simulink model "my"  (R2021a)
settings: Solver=VariableStepAuto  StartTime=0.0  StopTime=20  RelTol=1e-3
model workspace (MAT data in the model file):
  tc = 0.01
values from neighbouring files (symbols this model uses):
  cf = -155016    [emplanner_init.m]
  cr = -92204    [emplanner_init.m]
  la = 1.225    [emplanner_init.m]
  lb = 2.68-1.225    (= 1.455)    [emplanner_init.m]    (also in la3.m = -0.6; mpc_speed_control.m = kron(ones(Nc,1),-dumax))
  LQR_K1 = k(:,1)'    [emplanner_init.m]
  LQR_K2 = k(:,2)'    [emplanner_init.m]
  LQR_K3 = k(:,3)'    [emplanner_init.m]
  LQR_K4 = k(:,4)'    [emplanner_init.m]
  m = VehConf.m    [GetMPCControlMatrix.m]    (also in emplanner_init.m = 1422; getcontrol.m)
  vx_break_point = zeros(1,5000)    [emplanner_init.m]
libraries: simulink x3, pid_lib x2, Solver_SF x1
settings Model: Creator=t  LastModifiedBy=t

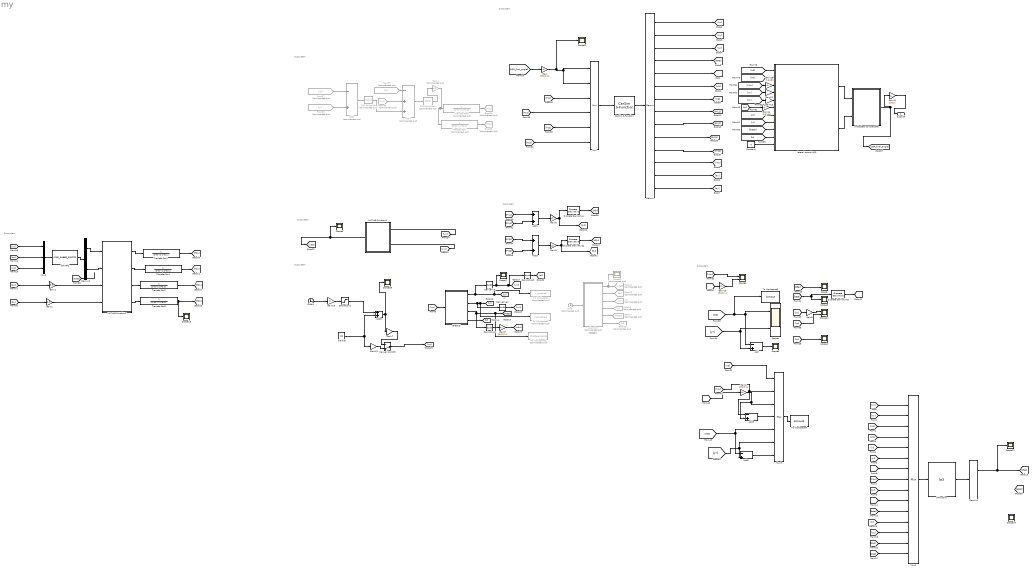
== system my ==
  note: Subsystem
  note: Subsystem
  note: Subsystem
  note: Subsystem
  note: Subsystem
  note: Subsystem
  note: 规划接口
  note: Subsystem
  Add : Sum  Inputs=-+
  Add1 : Sum
  Add2 : Sum  Commented=on  Inputs=-+
  Add3 : Sum
  Add4 : Sum  Commented=on  Inputs=-++
  Add5 : Sum  Inputs=-+
  Add6 : Sum  Inputs=-+
  Add8 : Sum
  CarSim S-Function : Solver_SF/CarSim S-Function  Priority=1  SIMFILE=simfile.sim  Run_RTs=off  vs_state_ind=Run  StopMode_ind=Vehicle Model
  Clock : Clock  Commented=on
  Clock1 : Clock
  Constant : Constant  Value=0
  Demux : Demux  Outputs=14
  Demux1 : Demux  Outputs=2
  Demux2 : Demux  Outputs=2
  Derivative{,1..3} (4 alike) : Derivative
  Discrete Derivative : simulink/Discrete/Discrete Derivative  gainval=1.0  ICPrevScaledInput=0.0  OutMin=[]  OutMax=[]  OutDataType=fixdt(1, 16)  OutScaling=2^-10  DoSatur=off
  Discrete Derivative1 : simulink/Discrete/Discrete Derivative  gainval=1.0  ICPrevScaledInput=0.0  OutMin=[]  OutMax=[]  OutDataType=fixdt(1, 16)  OutScaling=2^-10  DoSatur=off
  Discrete Derivative2 : simulink/Discrete/Discrete Derivative  gainval=1.0  ICPrevScaledInput=0.0  OutMin=[]  OutMax=[]  OutDataType=fixdt(1, 16)  OutScaling=2^-10  DoSatur=off
  From37 : From  Commented=on  GotoTag=xO
  From38 : From  Commented=on  GotoTag=xr
  From39 : From  Commented=on  GotoTag=Vx
  From46 : From  Commented=on  GotoTag=vp
  Gain{,3,6,10} (4 alike) : Gain  Gain=180/3.14
  Gain1 : Gain  Gain=9.8
  Gain11 : Gain  Gain=180/pi
  Gain{5,7,12..13,20} (5 alike) : Gain  Gain=1/3.6
  Gain14 : Gain  Gain=3.6/180
  Gain15 : Gain  Gain=3.6/180
  Gain19 : Gain  Gain=2
  Gain2 : Gain  Gain=9.8
  Gain4 : Gain  Commented=on  Gain=1/2
  Gain8 : Gain  Gain=1/2
  Gain9 : Gain  Gain=1/2
  Goto16 : Goto  Commented=on  GotoTag=yr
  Goto17 : Goto  Commented=on  GotoTag=thetar
  Goto18 : Goto  Commented=on  GotoTag=kr
  Goto24 : Goto  Commented=on  GotoTag=vdes
  Goto25 : Goto  Commented=on  GotoTag=ar
  Goto34 : Goto  Commented=on  GotoTag=T21
  Goto35 : Goto  Commented=on  GotoTag=T22
  MATLAB Function1 : MATLAB Function  TreatAsAtomicUnit=on
  MATLAB Function2 : MATLAB Function  TreatAsAtomicUnit=on
  Manual Switch5 : ManualSwitch  CurrentSetting=0
  Mux : Mux  Inputs=6
  Mux1 : Mux  Inputs=15
  Mux2 : Mux  Inputs=3
  Mux3 : Mux  Inputs=7
  PID Controller : pid_lib/PID Controller  Commented=on  Controller=PID  Form=Parallel  TimeDomain=Continuous-time  UseExternalTs=off  SampleTime=-1  IntegratorMethod=Forward Euler  FilterMethod=Forward Euler  ControllerParametersSource=internal  P=1  I=0.01  D=0  UseFilter=on  N=100  TunerSelectOption=Transfer Function Based (PID Tuner App)  InitialConditionSource=internal  InitialConditionForIntegrator=0  InitialConditionForFilter=0  DifferentiatorICPrevScaledInput=0  ExternalReset=none  TrackingMode=off  Kt=1  LimitOutput=off  SatLimitsSource=internal  UpperSaturationLimit=inf  LowerSaturationLimit=-inf  LinearizeAsGain=on  AntiWindupMode=none  Kb=1  POutMin=[]  POutMax=[]  IOutMin=[]  IOutMax=[]  DOutMin=[]  DOutMax=[]  NOutMin=[]  NOutMax=[]  SumOutMin=[]  SumOutMax=[]  SaturationOutMin=[]  SaturationOutMax=[]  PParamMin=[]  PParamMax=[]  IParamMin=[]  IParamMax=[]  DParamMin=[]  DParamMax=[]  NParamMin=[]  NParamMax=[]  KbParamMin=[]  KbParamMax=[]  KtParamMin=[]  KtParamMax=[]  KbOutMin=[]  KbOutMax=[]  KtOutMin=[]  KtOutMax=[]  IntegratorOutMin=[]  IntegratorOutMax=[]  FilterOutMin=[]  FilterOutMax=[]  SumI1OutMin=[]  SumI1OutMax=[]  SumI2OutMin=[]  SumI2OutMax=[]  SumI3OutMin=[]  SumI3OutMax=[]  SumI4OutMin=[]  SumI4OutMax=[]  SumDOutMin=[]  SumDOutMax=[]  DifferentiatorOutMin=[]  DifferentiatorOutMax=[]  FilterDiffOutCoefMin=[]  FilterDiffOutCoefMax=[]  ReciprocalOutMin=[]  ReciprocalOutMax=[]  SumDenOutMin=[]  SumDenOutMax=[]  SumNumOutMin=[]  SumNumOutMax=[]  DivideOutMin=[]  DivideOutMax=[]  UdiffTsProdOutMin=[]  UdiffTsProdOutMax=[]  NTsProdOutMin=[]  NTsProdOutMax=[]  UintegralTsProdOutMin=[]  UintegralTsProdOutMax=[]  UngainTsProdOutMin=[]  UngainTsProdOutMax=[]  IntegratorContinuousStateAttributes=''  IntegratorStateMustResolveToSignalObject=off  IntegratorRTWStateStorageClass=Auto  FilterContinuousStateAttributes=''  FilterStateMustResolveToSignalObject=off  FilterRTWStateStorageClass=Auto  ParallelPVariant=InternalParameters  IdealPVariant=Disabled  IVariant=InternalParameters  DVariant=InternalParameters  IntegratorVariant=Continuous  SatVariant=Disabled  AWVariant=Passthrough  PCopyVariant=Disabled  TRVariant=Disabled  FdbkBlocksVariant=Forward  IdealPFdbkVariant=Disabled  SatFdbkVariant=Disabled  DerivativeFilterVariant=ContFilter  NVariant=InternalParameters  NCopyVariant=Disabled  FilterICVariant=InternalICsFilter  IntegratorICVariant=InternalICs  ExternalResetVariant=Disabled  TRSumVariant=Passthrough  SumFdbkVariant=Disabled  SumVariant=Sum_PID  TsampFilterVariant=InternalTs  TsampNgainVariant=Passthrough  TsampIntegralVariant=Passthrough  ExternalSaturationOutDataTypeStr=Inherit: Same as second input
  PID Controller1 : pid_lib/PID Controller  Commented=on  Controller=PID  Form=Parallel  TimeDomain=Continuous-time  UseExternalTs=off  SampleTime=-1  IntegratorMethod=Forward Euler  FilterMethod=Forward Euler  ControllerParametersSource=internal  P=0.03  I=0.2  D=0  UseFilter=on  N=100  TunerSelectOption=Transfer Function Based (PID Tuner App)  InitialConditionSource=internal  InitialConditionForIntegrator=0  InitialConditionForFilter=0  DifferentiatorICPrevScaledInput=0  ExternalReset=none  TrackingMode=off  Kt=1  LimitOutput=off  SatLimitsSource=internal  UpperSaturationLimit=inf  LowerSaturationLimit=-inf  LinearizeAsGain=on  AntiWindupMode=none  Kb=1  POutMin=[]  POutMax=[]  IOutMin=[]  IOutMax=[]  DOutMin=[]  DOutMax=[]  NOutMin=[]  NOutMax=[]  SumOutMin=[]  SumOutMax=[]  SaturationOutMin=[]  SaturationOutMax=[]  PParamMin=[]  PParamMax=[]  IParamMin=[]  IParamMax=[]  DParamMin=[]  DParamMax=[]  NParamMin=[]  NParamMax=[]  KbParamMin=[]  KbParamMax=[]  KtParamMin=[]  KtParamMax=[]  KbOutMin=[]  KbOutMax=[]  KtOutMin=[]  KtOutMax=[]  IntegratorOutMin=[]  IntegratorOutMax=[]  FilterOutMin=[]  FilterOutMax=[]  SumI1OutMin=[]  SumI1OutMax=[]  SumI2OutMin=[]  SumI2OutMax=[]  SumI3OutMin=[]  SumI3OutMax=[]  SumI4OutMin=[]  SumI4OutMax=[]  SumDOutMin=[]  SumDOutMax=[]  DifferentiatorOutMin=[]  DifferentiatorOutMax=[]  FilterDiffOutCoefMin=[]  FilterDiffOutCoefMax=[]  ReciprocalOutMin=[]  ReciprocalOutMax=[]  SumDenOutMin=[]  SumDenOutMax=[]  SumNumOutMin=[]  SumNumOutMax=[]  DivideOutMin=[]  DivideOutMax=[]  UdiffTsProdOutMin=[]  UdiffTsProdOutMax=[]  NTsProdOutMin=[]  NTsProdOutMax=[]  UintegralTsProdOutMin=[]  UintegralTsProdOutMax=[]  UngainTsProdOutMin=[]  UngainTsProdOutMax=[]  IntegratorContinuousStateAttributes=''  IntegratorStateMustResolveToSignalObject=off  IntegratorRTWStateStorageClass=Auto  FilterContinuousStateAttributes=''  FilterStateMustResolveToSignalObject=off  FilterRTWStateStorageClass=Auto  ParallelPVariant=InternalParameters  IdealPVariant=Disabled  IVariant=InternalParameters  DVariant=InternalParameters  IntegratorVariant=Continuous  SatVariant=Disabled  AWVariant=Passthrough  PCopyVariant=Disabled  TRVariant=Disabled  FdbkBlocksVariant=Forward  IdealPFdbkVariant=Disabled  SatFdbkVariant=Disabled  DerivativeFilterVariant=ContFilter  NVariant=InternalParameters  NCopyVariant=Disabled  FilterICVariant=InternalICsFilter  IntegratorICVariant=InternalICs  ExternalResetVariant=Disabled  TRSumVariant=Passthrough  SumFdbkVariant=Disabled  SumVariant=Sum_PID  TsampFilterVariant=InternalTs  TsampNgainVariant=Passthrough  TsampIntegralVariant=Passthrough  ExternalSaturationOutDataTypeStr=Inherit: Same as second input
  S-Function : S-Function  FunctionName=la3  SFunctionDeploymentMode=off  EnableBusSupport=off
  Saturation1 : Saturate  UpperLimit=18  LowerLimit=-18
  Scope{,1,3,5..8,10,12..13,28} (11 alike) : Scope
  Scope11 : Scope  NumInputPorts=2
  Scope2 : Scope  NumInputPorts=2
  Scope4 : Scope  NumInputPorts=2
  Scope9 : Scope  Commented=on
  To Workspace : ToWorkspace  Commented=on  VariableName=x_experice  SaveFormat=Timeseries  SampleTime=-1
  To Workspace1 : ToWorkspace  Commented=on  VariableName=y_experice1  SaveFormat=Timeseries  SampleTime=-1
  To Workspace2 : ToWorkspace  Commented=on  VariableName=theate_experice  SaveFormat=Timeseries  SampleTime=-1
  To Workspace3 : ToWorkspace  VariableName=simout  SaveFormat=Timeseries  SampleTime=-1
  To Workspace4 : ToWorkspace  VariableName=simout1  SaveFormat=Timeseries  SampleTime=-1
  Transfer Fcn{1..4} (4 alike) : TransferFcn  Denominator=[2*tc^2 2*tc 1]
  Transfer Fcn6 : TransferFcn  Commented=on  Denominator=[2*tc^2 2*tc 1]
  Transfer Fcn7 : TransferFcn  Commented=on  Denominator=[2*tc^2 2*tc 1]
  lateral control LQR : Subsystem
  planning : MATLAB Function  Commented=on  TreatAsAtomicUnit=on
  understeer compensate : Subsystem
  xr1 : Goto  Commented=on  GotoTag=xr
  参考轨迹 : Subsystem
  目标车速 : Constant  Value=60
  纵向MPC : S-Function  FunctionName=mpc_speed_control  SFunctionDeploymentMode=off  EnableBusSupport=off
  Output3 : Outport
  wires:
  ? -> [ades], Scope10/1
  planning/6(kr) -> Goto18/1  "曲率"
  [xO] -> lateral control LQR/1(host_x[m])
  Demux/7 -> [YO]
  [yr] -> lateral control LQR/8(yr)
  [ax] -> Gain1/1
  Gain14/1 -> lateral control LQR/6(host_yaw_dot[rad/s])
  lateral control LQR/1(Output) -> understeer compensate/1(LQR_angle)
  Transfer Fcn4/1 -> [T11]
  Add4/1 -> PID Controller1/1
  Gain12/1 -> lateral control LQR/4(host_vx[m/s])
  Discrete Derivative1/1 -> [dfyr]
  [Vx] -> Gain12/1
  [vp] -> Scope11/2
  [bata] -> Mux1/11
  Gain10/1 -> Scope2/2
  PID Controller1/1 -> Gain4/1
  PID Controller/1 -> Add4/3
  [CAF] -> Mux1/14
  [FYL1] -> Add1/1
  [kr] -> lateral control LQR/10(kappar)
  Demux/8 -> [FYL1]  "FYL1"
  Add2/1 -> PID Controller/1
  From39/1 -> Add4/1
  MATLAB Function2/4(T22) -> Transfer Fcn3/1
  From38/1 -> Add2/2
  Derivative3/1 -> [ar]
  From46/1 -> Add4/2
  From37/1 -> Add2/1
  Gain1/1 -> MATLAB Function2/3(ax)
  Demux/14 -> [ay]  "横向加速度"
  [LQR_final_angle] -> Gain/1  "转角"
  Demux/3 -> [wr]  "横摆角速度deg/s"
  [wr] -> Mux1/9
  [yr] -> Add/2, Scope4/2
  [xr] -> Mux1/5
  lateral control LQR/2(Output1) -> understeer compensate/2(lateral err)
  [T11] -> Mux/3
  [YO] -> To Workspace3/1, Scope4/1, Add/1
  Demux/12 -> [YAw]  "ya(deg)"
  [T22] -> Mux/6
  [dbate] -> Mux1/10
  [YAw] -> Mux1/8
  Demux/1 -> [Vx]  "vx(km/h)"
  [T12] -> Mux/4
  [vp] -> Mux2/3
  [Vx] -> Gain5/1
  Gain3/1 -> [wthr]
  [stter] -> Scope/1
  [wr] -> Scope1/1
  Transfer Fcn2/1 -> [T21]
  Mux2/1 -> 纵向MPC/1
  MATLAB Function2/1(T11) -> Transfer Fcn4/1
  目标车速/1 -> Gain20/1, Add8/2
  Gain20/1 -> Manual Switch5/2
  Clock1/1 -> Gain19/1
  参考轨迹/3(yawr) -> Derivative2/1, To Workspace2/1, [thetar]  "yawa"
  planning/4(yr) -> Goto16/1
  Gain19/1 -> Saturation1/1
  Saturation1/1 -> Add8/1
  Manual Switch5/1 -> [vp]
  Gain7/1 -> Manual Switch5/1
  Add8/1 -> Gain7/1, Scope28/1
  planning/2(ap) -> Goto25/1  "ap"
  [ades] -> ?
  参考轨迹/2(yr) -> Derivative1/1, To Workspace1/1, [yr]
  MATLAB Function2/3(T21) -> Transfer Fcn2/1
  Demux/6 -> [xO]
  Transfer Fcn1/1 -> [T12]
  [kr] -> Mux1/12
  Mux/1 -> CarSim S-Function/1
  Mux1/1 -> S-Function/1
  Demux/2 -> [Vy]  "vy"
  [bata] -> Scope3/1, Discrete Derivative2/1
  planning/1(vp) -> Scope9/1, Goto24/1  "vp"
  Add/1 -> Scope5/1
  Demux/13 -> [ax]  "纵向加速度"
  MATLAB Function1/1(v) -> Scope6/1, [vact]
  参考轨迹/1(xr) -> Derivative/1, To Workspace/1, [xr]
  参考轨迹/4(kr) -> [kr]  "曲率"
  Gain9/1 -> [fyr], Discrete Derivative1/1
  planning/5(thetar) -> Goto17/1  "a"
  [YAw] -> Scope2/1
  MATLAB Function2/2(T12) -> Transfer Fcn1/1
  Transfer Fcn7/1 -> Goto35/1
  [YO] -> lateral control LQR/2(host_y[m])
  Constant/1 -> lateral control LQR/11(predict_time)
  [ax] -> Mux2/2
  [YAw] -> Gain15/1
  Demux1/1 -> [stter], Scope12/1
  [FYR1] -> Add3/1
  [vyr] -> MATLAB Function1/2(vy)
  [thetar] -> Gain10/1
  Discrete Derivative2/1 -> [dbate]
  [Vx] -> Mux1/1
  Gain4/1 -> Transfer Fcn7/1, Transfer Fcn6/1
  Gain11/1 -> Output3/1
  [vp] -> Mux1/13
  [xr] -> lateral control LQR/7(xr)
  Demux2/1 -> MATLAB Function2/1(Vx)
  Demux/5 -> [ster_L]
  Demux/10 -> [FYR1]  "FYR1"
  Add1/1 -> Gain8/1
  Add3/1 -> Gain9/1
  understeer compensate/1(LQR_final_angle) -> [LQR_final_angle], Gain11/1
  [thetar] -> lateral control LQR/9(thetar)
  Transfer Fcn3/1 -> [T22], Scope13/1
  Transfer Fcn6/1 -> Goto34/1
  [YO] -> Mux1/3
  [vp] -> 参考轨迹/1(vx)
  [CAR] -> Mux1/15
  [FYL2] -> Add1/2
  [ay] -> Gain2/1
  Gain5/1 -> Scope11/1
  [Vy] -> Mux1/2
  [Vx] -> Mux2/1
  Clock/1 -> planning/1(t)
  planning/3(xr) -> xr1/1
  [thetar] -> Mux1/7
  Demux/9 -> [FYL2]  "FYL2"
  [yr] -> Mux1/6
  Demux/11 -> [FYR2]  "FYR2"
  Gain/1 -> Scope8/1, Mux/1, Mux/2
  Gain2/1 -> MATLAB Function2/4(ay)
  Gain8/1 -> Discrete Derivative/1, [fyf]
  Discrete Derivative/1 -> [dfyf]
  Derivative1/1 -> [vyr]
  [vxr] -> MATLAB Function1/1(vx)
  Derivative2/1 -> Gain3/1
  Derivative/1 -> Derivative3/1, [vxr], Scope7/1
  Demux/4 -> [bata]  "质心侧偏角(deg)"
  [T21] -> Mux/5
  Demux2/2 -> MATLAB Function2/2(adex)
  [Vy] -> Gain13/1
  S-Function/1 -> Demux1/1
  [xO] -> Mux1/4
  Gain15/1 -> lateral control LQR/3(host_yaw[rad])
  纵向MPC/1 -> Demux2/1
  [FYR2] -> Add3/2
  Gain13/1 -> lateral control LQR/5(host_vy[m/s])
  CarSim S-Function/1 -> Demux/1
  [wr] -> Gain14/1
  Mux3/1 -> To Workspace4/1
  [thetar] -> Gain6/1
  [YAw] -> Mux3/2, Add5/1  "实际航向角"
  Gain6/1 -> Add5/2, Mux3/3  "理想航向角"
  [YO] -> Mux3/5, Add6/1  "实际横向"
  [yr] -> Mux3/6, Add6/2  "理想横向"
  Add5/1 -> Mux3/4  "航向偏差"
  Add6/1 -> Mux3/7  "横向偏差"
  [xO] -> Mux3/1

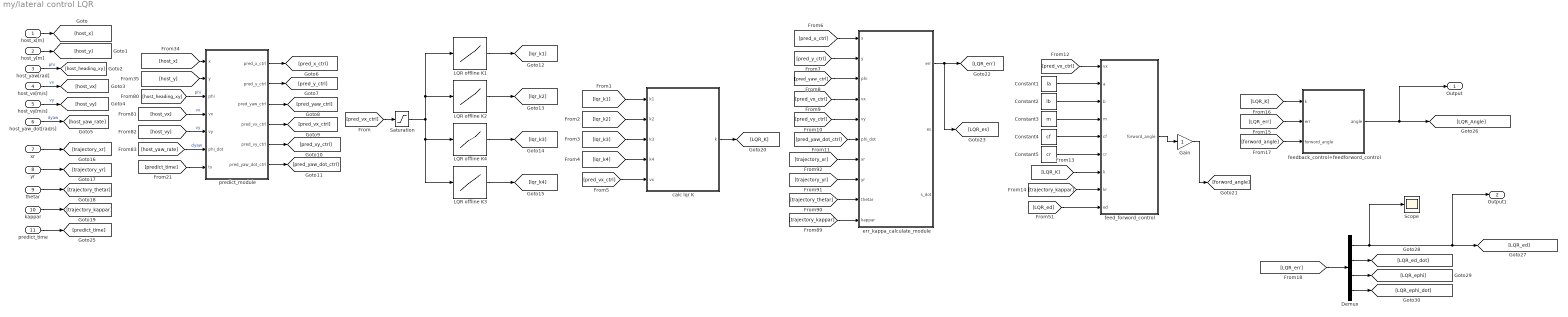
== system my/lateral control LQR ==
  host_x[m] : Inport
  host_y[m] : Inport  Port=2
  host_yaw[rad] : Inport  Port=3
  host_vx[m/s] : Inport  Port=4
  host_vy[m/s] : Inport  Port=5
  host_yaw_dot[rad/s] : Inport  Port=6
  xr : Inport  Port=7
  yr : Inport  Port=8
  thetar : Inport  Port=9
  kappar : Inport  Port=10
  predict_time : Inport  Port=11
  Constant1 : Constant  Value=la
  Constant2 : Constant  Value=lb
  Constant3 : Constant  Value=m
  Constant4 : Constant  Value=cf
  Constant5 : Constant  Value=cr
  Demux : Demux
  Gain : Gain
  LQR offline K1 : Lookup_n-D  NumberOfTableDimensions=1  BreakpointsForDimension1=vx_break_point  Table=LQR_K1  InternalRulePriority=Speed  RndMeth=Simplest  InputSameDT=on
  LQR offline K2 : Lookup_n-D  NumberOfTableDimensions=1  BreakpointsForDimension1=vx_break_point  Table=LQR_K2  InternalRulePriority=Speed  RndMeth=Simplest  InputSameDT=on
  LQR offline K3 : Lookup_n-D  NumberOfTableDimensions=1  BreakpointsForDimension1=vx_break_point  Table=LQR_K3  InternalRulePriority=Speed  RndMeth=Simplest  InputSameDT=on
  LQR offline K4 : Lookup_n-D  NumberOfTableDimensions=1  BreakpointsForDimension1=vx_break_point  Table=LQR_K4  InternalRulePriority=Speed  RndMeth=Simplest  InputSameDT=on
  Saturation : Saturate  UpperLimit=50  LowerLimit=0
  Scope : Scope
  calc lqr K : MATLAB Function  TreatAsAtomicUnit=on
  err_kappa_calculate_module : MATLAB Function  TreatAsAtomicUnit=on
  feed_forword_control : MATLAB Function  TreatAsAtomicUnit=on
  feedback_control+feedforword_control : MATLAB Function  TreatAsAtomicUnit=on
  predict_module : MATLAB Function  TreatAsAtomicUnit=on
  Output : Outport
  Output1 : Outport  Port=2
  wires:
  [host_vy] -> predict_module/5(vy)  "vy"
  [host_x] -> predict_module/1(x)
  [host_yaw_rate] -> predict_module/6(phi_dot)  "dyaw"
  [host_vx] -> predict_module/4(vx)  "vx"
  [host_y] -> predict_module/2(y)
  [host_heading_xy] -> predict_module/3(phi)  "phi"
  [predict_time] -> predict_module/7(ts)
  host_x[m]/1 -> [host_x]
  host_y[m]/1 -> [host_y]
  host_yaw[rad]/1 -> [host_heading_xy]  "phi"
  host_vx[m/s]/1 -> [host_vx]  "vx"
  host_vy[m/s]/1 -> [host_vy]  "vy"
  host_yaw_dot[rad/s]/1 -> [host_yaw_rate]  "dyaw"
  predict_module/1(pred_x_ctrl) -> [pred_x_ctrl]
  predict_module/2(pred_y_ctrl) -> [pred_y_ctrl]
  predict_module/3(pred_yaw_ctrl) -> [pred_yaw_ctrl]
  predict_module/4(pred_vx_ctrl) -> [pred_vx_ctrl]
  predict_module/5(pred_vy_ctrl) -> [pred_vy_ctrl]
  predict_module/6(pred_yaw_dot_ctrl) -> [pred_yaw_dot_ctrl]
  [pred_vx_ctrl] -> Saturation/1
  LQR offline K1/1 -> [lqr_k1]
  LQR offline K2/1 -> [lqr_k2]
  LQR offline K4/1 -> [lqr_k3]
  LQR offline K3/1 -> [lqr_k4]
  [pred_vx_ctrl] -> calc lqr K/5(vx)
  [lqr_k4] -> calc lqr K/4(k4)
  [lqr_k3] -> calc lqr K/3(k3)
  [lqr_k2] -> calc lqr K/2(k2)
  [lqr_k1] -> calc lqr K/1(k1)
  [pred_x_ctrl] -> err_kappa_calculate_module/1(x)
  [pred_y_ctrl] -> err_kappa_calculate_module/2(y)
  [pred_yaw_ctrl] -> err_kappa_calculate_module/3(phi)
  [pred_vx_ctrl] -> err_kappa_calculate_module/4(vx)
  [pred_vy_ctrl] -> err_kappa_calculate_module/5(vy)
  [pred_yaw_dot_ctrl] -> err_kappa_calculate_module/6(phi_dot)
  xr/1 -> [trajectory_xr]
  yr/1 -> [trajectory_yr]
  thetar/1 -> [trajectory_thetar]
  kappar/1 -> [trajectory_kappar]
  [trajectory_xr] -> err_kappa_calculate_module/7(xr)
  [trajectory_yr] -> err_kappa_calculate_module/8(yr)
  [trajectory_kappar] -> err_kappa_calculate_module/10(kappar)
  [trajectory_thetar] -> err_kappa_calculate_module/9(thetar)
  [pred_vx_ctrl] -> feed_forword_control/1(vx)
  Constant1/1 -> feed_forword_control/2(a)
  Constant2/1 -> feed_forword_control/3(b)
  Constant3/1 -> feed_forword_control/4(m)
  Constant4/1 -> feed_forword_control/5(cf)
  Constant5/1 -> feed_forword_control/6(cr)
  calc lqr K/1(k) -> [LQR_K]
  [LQR_K] -> feed_forword_control/7(k)
  [trajectory_kappar] -> feed_forword_control/8(kr)
  feed_forword_control/1(forword_angle) -> Gain/1
  [LQR_err] -> feedback_control+feedforword_control/2(err)
  [LQR_K] -> feedback_control+feedforword_control/1(k)
  [forword_angle] -> feedback_control+feedforword_control/3(forword_angle)
  [LQR_err] -> Demux/1
  err_kappa_calculate_module/1(err) -> [LQR_es], [LQR_err]
  Saturation/1 -> LQR offline K3/1, LQR offline K4/1, LQR offline K2/1, LQR offline K1/1
  predict_time/1 -> [predict_time]
  feedback_control+feedforword_control/1(angle) -> Output/1, [LQR_Angle]
  Demux/1 -> Scope/1, Output1/1, [LQR_ed]
  Demux/2 -> [LQR_ed_dot]
  Demux/3 -> [LQR_ephi]
  Demux/4 -> [LQR_ephi_dot]
  [LQR_ed] -> feed_forword_control/9(ed)
  Gain/1 -> [forword_angle]

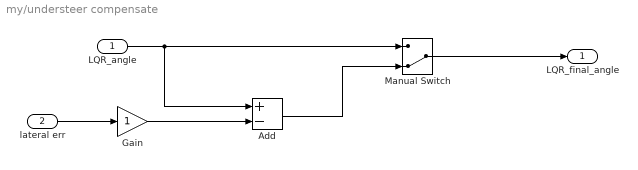
== system my/understeer compensate ==
  LQR_angle : Inport
  lateral err : Inport  Port=2
  Add : Sum  Inputs=+-
  Gain : Gain
  Manual Switch : ManualSwitch  CurrentSetting=0
  LQR_final_angle : Outport
  wires:
  Add/1 -> Manual Switch/2
  Manual Switch/1 -> LQR_final_angle/1
  LQR_angle/1 -> Add/1, Manual Switch/1
  lateral err/1 -> Gain/1
  Gain/1 -> Add/2

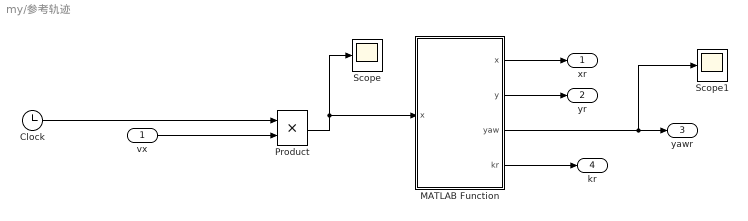
== system my/参考轨迹 ==
  vx : Inport
  Clock : Clock
  MATLAB Function : MATLAB Function  TreatAsAtomicUnit=on
  Product : Product
  Scope : Scope
  Scope1 : Scope
  xr : Outport
  yr : Outport  Port=2
  yawr : Outport  Port=3
  kr : Outport  Port=4
  wires:
  MATLAB Function/1(x) -> xr/1
  MATLAB Function/2(y) -> yr/1
  MATLAB Function/3(yaw) -> Scope1/1, yawr/1
  Clock/1 -> Product/1
  vx/1 -> Product/2
  Product/1 -> MATLAB Function/1("x "), Scope/1
  MATLAB Function/4(kr) -> kr/1

== matlab function my/lateral control LQR/feedback_control+feedforword_control ==
  data: k input; angle output; err input; forword_angle input
function angle = fcn(k,err,forword_angle)

    angle=-k*err+forword_angle;
    %angle=-k*err;
end

== matlab function my/lateral control LQR/calc lqr K ==
  data: k1 input; k output; k2 input; k3 input; k4 input; vx input
function k  = fcn(k1,k2,k3,k4,vx)
    if abs(vx)<0.1
        k=[0,0,0,0];
    else
       
        k=[k1,k2,k3,k4];
    end
end

== matlab function my/lateral control LQR/predict_module ==
  data: x input; pred_x_ctrl output; y input; phi input; vx input; vy input; phi_dot input; ts input; pred_y_ctrl output; pred_yaw_ctrl output; pred_vx_ctrl output; pred_vy_ctrl output; pred_yaw_dot_ctrl output
function [pred_x_ctrl,pred_y_ctrl,pred_yaw_ctrl,pred_vx_ctrl,pred_vy_ctrl,pred_yaw_dot_ctrl] = fcn(x,y,phi,vx,vy,phi_dot,ts)
    pred_x_ctrl=x+vx*ts*cos(phi)-vy*ts*sin(phi);
    pred_y_ctrl=y+vy*ts*cos(phi)+vx*ts*sin(phi);
    pred_yaw_ctrl=phi;
    pred_vx_ctrl=vx;
    pred_vy_ctrl=vy;
    pred_yaw_dot_ctrl=phi_dot;
end

== matlab function my/参考轨迹/MATLAB Function ==
  data: x output; y output; x input; yaw output; kr output
function [x,y,yaw,kr] = fcn(x)
%SUNZHE双移线

% r1=0.096*(x-60)-1.2;
% r2=0.096*(x-120)-1.2;
% dm1=25;
% dm2=25;
% dn1=3.6;
% dn2=3.6;
% y = dn1/2*(1+tanh(r1))-dn2/2*(1+tanh(r2));
% yaw = atan(dn1*(1/cosh(r1))^2*(1.2/dm1)-dn2*(1/cosh(r2))^2*(1.2/dm2));
% %plot(x,y)
% %y'
% y1=(108*tanh((12*x)/125 - 318/25)^2)/625 - (108*tanh((12*x)/125 - 174/25)^2)/625;
% %
% y2=(216*tanh((12*x)/125 - 174/25)*((12*tanh((12*x)/125 - 174/25)^2)/125 - 12/125))/625 - (216*tanh((12*x)/125 - 318/25)*((12*tanh((12*x)/125 - 318/25)^2)/125 - 12/125))/625;
% kr=y2/(1+(y1)^2)^(3/2);
% 


%%%%%%%%%%%%%%%
%mpc书上双移线
dx1=25;
dx2=21.95;
dy1=4.05;
dy2=5.7;
z11=2.4/25*(x-27.19)-1.2;
z12=2.4/21.95*(x-56.46)-1.2;
y=dy1/2*(1+tanh(z11))-dy2/2*(1+tanh(z12));
yaw=atan(dy1*(1/cosh(z11))^2*(1.2/dx1)-dy2*(1/cosh(z12))^2*(1.2/dx2));
y1=(684*tanh((48*x)/439 - 80922/10975)^2)/2195 - (243*tanh((12*x)/125 - 11907/3125)^2)/1250 - 64323/548750;
y2=(243*tanh((12*x)/125 - 11907/3125)*((12*tanh((12*x)/125 - 11907/3125)^2)/125 - 12/125))/625 - (1368*tanh((48*x)/439 - 80922/10975)*((48*tanh((48*x)/439 - 80922/10975)^2)/439 - 48/439))/2195;
kr=y2/(1+(y1)^2)^(3/2);

== matlab function my/MATLAB Function1 ==
  data: vx input; v output; vy input
function v = fcn(vx,vy)
v=sqrt(vx^2+vy^2);
end

== matlab function my/planning ==
  data: vp output; ap output; t input; xr output; yr output; thetar output; kr output
function [vp,ap,xr,yr,thetar,kr] = fcn(t)
    dx=100;
    dy=10;
    T=80;
    xstart=[0,0,0];
    xend=[dx,0,0];
    ystart=[0,0,0];
    yend=[dy,0,0];
    a=zeros(1,6);
    b=zeros(1,6);
    
    a(1)=xstart(1);
    a(2)=xstart(2);
    a(3)=xstart(3)/2;
    A1=[T^3,T^4,T^5;
        3*T^2,4*T^3,5*T^4;
        6*T,12*T^2,20*T^3];
    B1=[xend(1)-a(1)-a(2)*T-a(3)*T^2;
        xend(2)-a(2)-2*a(3)*T;
        xend(3)-2*a(3)];
    xs=inv(A1)*B1;
    a(4)=xs(1);
    a(5)=xs(2);
    a(6)=xs(3);
    b(1)=ystart(1);
    b(2)=ystart(2);
    b(3)=ystart(3)/2;
    A2=[dx^3,dx^4,dx^5;
        3*dx^2,4*dx^3,5*dx^4;
        6*dx,12*dx^2,20*dx^3];
    B2=[yend(1)-b(1)-b(2)*dx-b(3)*dx^2;
        yend(2)-b(2)-2*b(3)*dx;
        yend(3)-2*b(3)];
    ys=inv(A2)*B2;
    b(4)=ys(1);
    b(5)=ys(2);
    b(6)=ys(3);
    xr=a(1)+a(2)*t+a(3)*t^2+a(4)*t^3+a(5)*t^4+a(6)*t^5;
    yr=b(1)+b(2)*xr+b(3)*xr^2+b(4)*xr^3+b(5)*xr^4+b(6)*xr^5;
    xr_dot=a(2)+2*a(3)*t+3*a(4)*t^2+4*a(5)*t^3+5*a(6)*t^4;
    yr_dx=b(2)+2*b(3)*xr+3*b(4)*xr^2+4*b(5)*xr^3+5*b(6)*xr^4;
    yr_dot=yr_dx*xr_dot;
    thetar=atan(yr_dx);
    xr_dot2=2*a(3)+6*a(4)*t+12*a(5)*t^2+20*a(6)*t^3;
    yr_dx2=2*b(3)+6*b(4)*xr+12*b(5)*xr^2+20*b(6)*xr^3;
    yr_dot2=yr_dx2*xr_dot^2+yr_dx*xr_dot2;
    kr=yr_dx2/((1+yr_dx^2)^1.5);
    vp=sqrt(xr_dot^2+yr_dot^2);
    if xr_dot2>=0
        ap=sqrt(xr_dot2^2+yr_dot2^2);
    else
        ap=-sqrt(xr_dot2^2+yr_dot2^2);
    end

== matlab function my/MATLAB Function2 ==
  data: Vx input; adex input; T11 output; T12 output; T21 output; T22 output; ax input; ay input
function [T11,T12,T21,T22] = fcn(Vx,adex,ax,ay)
A=0.3;
Cd=2.2;
f=0.005;
yita=0.95;
Vx=Vx*3.6;
m=1270+88+54;%整车质量
a=1.225;%质心到前轴的距离
b=2.68-1.22;%质心到后轴的距离
Bf=1.675;%前轴轮距
Br=1.675;%后轴轮距
r=0.325;%轮胎有效滚动半径
hg=0.54;%质心里地面高度
L=2.68;%轴距
g=9.8;%重力加速度
if(adex<0)
T_F=-1*(m*g*f+Cd*A/21.15*Vx^2+m*adex)*0.325/yita;
else
T_F=(m*g*f+Cd*A/21.15*Vx^2+m*adex)*0.325/yita;
end
    
%% 计算各个车轮力矩
Fz11=m*g*b/2/L-m*ax*hg/2/L-m*ay*b*hg/L/Bf;
Fz12=m*g*b/2/L-m*ax*hg/2/L+m*ay*b*hg/L/Bf;
Fz21=m*g*a/2/L+m*ax*hg/2/L-m*ay*a*hg/L/Br;
Fz22=m*g*a/2/L+m*ax*hg/2/L+m*ay*a*hg/L/Br;

T11d=Fz11/(Fz11+Fz12+Fz21+Fz22)*(T_F);
T12d=Fz12/(Fz11+Fz12+Fz21+Fz22)*(T_F);
T21d=Fz21/(Fz11+Fz12+Fz21+Fz22)*(T_F);
T22d=Fz22/(Fz11+Fz12+Fz21+Fz22)*(T_F);

miu=1;
%左前轮
if  T11d>=miu*Fz11*r
    T11=miu*Fz11;
elseif  T11d<=-miu*Fz11*r
    T11=-miu*Fz11;
else
    T11=T11d;
end
%右前轮
if  T12d>=miu*Fz12*r
    T12=miu*Fz12;
elseif  T12d<=-miu*Fz12*r
    T12=-miu*Fz12;
else
    T12=T12d;
end
%左后轮
if  T21d>=miu*Fz21*r
    T21=miu*Fz21;
elseif  T21d<=-miu*Fz21*r
    T21=-miu*Fz21;
else
    T21=T21d;
end
%右后轮
if  T22d>=miu*Fz22*r
    T22=miu*Fz22;
elseif  T22d<=-miu*Fz22*r
    T22=-miu*Fz22;
else
    T22=T22d;
end

== matlab function my/lateral control LQR/err_kappa_calculate_module ==
  data: x input; y input; phi input; vx input; vy input; phi_dot input; xr input; yr input; thetar input; kappar input; err output; es output; s_dot output
function [err ,es,s_dot]  = fcn(x,y,phi,vx,vy,phi_dot,xr,yr,thetar,kappar)
    

   
    tor=[cos(thetar);sin(thetar)];
    nor=[-sin(thetar);cos(thetar)];
    d_err=[x-xr;y-yr];
    ed=nor'*d_err;
    es=tor'*d_err;
     %projection_point_thetar=thetar(dmin);%apollo
    projection_point_thetar=thetar+kappar*es;
    ed_dot=vy*cos(phi-projection_point_thetar)+vx*sin(phi-projection_point_thetar);
    %%%%%%%%%
    ephi=sin(phi-projection_point_thetar);
    %%%%%%%%%
    ss_dot=vx*cos(phi-projection_point_thetar)-vy*sin(phi-projection_point_thetar);
    s_dot=ss_dot/(1-kappar*ed);
    ephi_dot=phi_dot-kappar*s_dot; 

%论文误差
%     ed=(y-yr)*cos(phi-thetar)-(x-xr)*sin(phi-thetar);
%     ed_dot=vx*sin(phi-thetar)+vy*cos(phi-thetar);
%     ephi=phi-thetar;
%     ephi_dot=phi_dot-vx*kappar;
    
    
    
    err=[ed;ed_dot;ephi;ephi_dot];
    
    
    
    
    
    
    
    
    
    
    
    


end

== matlab function my/lateral control LQR/feed_forword_control ==
  data: vx input; a input; forword_angle output; b input; m input; cf input; cr input; k input; kr input; ed input
function forword_angle = fcn(vx,a,b,m,cf,cr,k,kr,ed)
%为何支取前三位
% k 离线lqr
    forword_angle=kr*(a+b-b*k(3)-(m*vx*vx/(a+b))*((b/cf)+(a/cr)*k(3)-(a/cr)));
    %forword_angle=kr*(a+b-b*k(3)-(m*vx*vx/(a+b))*((b/cf/(1+abs(ed)))+(a/cr/(1+abs(ed)))*k(3)-(a/cr/(1+abs(ed)))));
end
